simulink model "ADK_signal_transfer"  (R2021a)
settings: configuration reference "ADK_IDS_Speedgoat" (kept outside this file)
undefined symbols (not defined in the file): COMMUNICATION_CYCLE_TIME, desired_trajectory_index, GNSS_Status, h, km, m, MAX_LOCAL_TRAJECTORY_WAY_POINT_NUMBER, MAX_TRAJECTORY_WAY_POINT_NUMBER, O_ALTITUDE, O_LATITUDE, O_LONGITUDE, s
libraries: simulink x3, simulink_extras x2, aerolibconvert2 x1
settings Model: DataDictionary=ADK_IDS.sldd  Creator=xinrui  LastModifiedBy=Administrator
settings ConfigSetRef: SourceName=ADK_IDS_Speedgoat

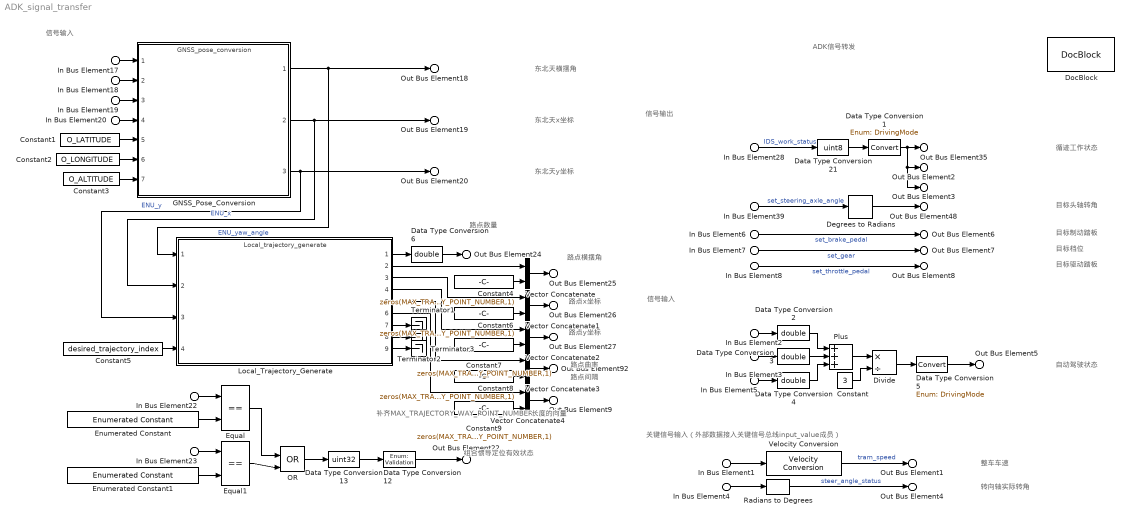
== system ADK_signal_transfer ==
  note: 信号输入
  note: 信号输出
  note: 信号输入
  note: 整车车速
  note: 关键信号输入（外部数据接入关键信号总线input_value成员）
  note: 转向轴实际转角
  note: 东北天横摆角
  note: 东北天x坐标
  note: 东北天y坐标
  note: 组合惯导定位有效状态
  note: 路点数量
  note: 路点横摆角
  note: 路点x坐标
  note: 路点y坐标
  note: 循迹工作状态
  note: 目标头轴转角
  note: 路点曲率
  note: 自动驾驶状态
  note: 目标制动踏板
  note: 目标档位
  note: 目标驱动踏板
  note: ADK信号转发
  note: 补齐MAX_TRAJECTORY_WAY_POINT_NUMBER长度的向量
  note: 路点间隔
  In Bus Element28 : Inport  PortName=IDS_InternalOutputPort  Element=IDS_work_status
  In Bus Element39 : Inport  PortName=IDS_InternalOutputPort  Element=steering_axle_info.set_angle.processed_value_current
  In Bus Element6 : Inport  PortName=IDS_InternalOutputPort  Element=AION_longitudinal_control_info.set_brake_pedal
  In Bus Element7 : Inport  PortName=IDS_InternalOutputPort  Element=AION_longitudinal_control_info.set_gear
  In Bus Element8 : Inport  PortName=IDS_InternalOutputPort  Element=AION_longitudinal_control_info.set_throttle_pedal
  In Bus Element2 : Inport  Port=2  PortName=IDS_InputPort  Element=InputCAN_bus.VCU2IDS_bus.VCU2IDS_brake_status.brake_pedal_enable_status
  In Bus Element1 : Inport  Port=2  PortName=IDS_InputPort  Element=InputCAN_bus.VCU2IDS_bus.VCU2IDS_status1.vehicle_speed
  In Bus Element3 : Inport  Port=2  PortName=IDS_InputPort  Element=InputCAN_bus.VCU2IDS_bus.VCU2IDS_steer_status.steer_angle_enable_status
  In Bus Element4 : Inport  Port=2  PortName=IDS_InputPort  Element=InputCAN_bus.VCU2IDS_bus.VCU2IDS_steer_status.steer_angle_status
  In Bus Element5 : Inport  Port=2  PortName=IDS_InputPort  Element=InputCAN_bus.VCU2IDS_bus.VCU2IDS_throttle_status.throttle_pedal_enable_status
  In Bus Element17 : Inport  Port=2  PortName=IDS_InputPort  Element=InputSerial_bus.GNSS2IDS_bus.Heading
  In Bus Element18 : Inport  Port=2  PortName=IDS_InputPort  Element=InputSerial_bus.GNSS2IDS_bus.Latitude
  In Bus Element19 : Inport  Port=2  PortName=IDS_InputPort  Element=InputSerial_bus.GNSS2IDS_bus.Longitude
  In Bus Element20 : Inport  Port=2  PortName=IDS_InputPort  Element=InputSerial_bus.GNSS2IDS_bus.Altitude
  In Bus Element22 : Inport  Port=2  PortName=IDS_InputPort  Element=InputSerial_bus.GNSS2IDS_bus.GNSSWorkStatus
  In Bus Element23 : Inport  Port=2  PortName=IDS_InputPort  Element=InputSerial_bus.GNSS2IDS_bus.GNSSWorkStatus
  Constant : Constant  Value=3
  Constant1 : Constant  Value=O_LATITUDE  OutDataTypeStr=double  SampleTime=COMMUNICATION_CYCLE_TIME
  Constant2 : Constant  Value=O_LONGITUDE  OutDataTypeStr=double  SampleTime=COMMUNICATION_CYCLE_TIME
  Constant3 : Constant  Value=O_ALTITUDE  OutDataTypeStr=double  SampleTime=COMMUNICATION_CYCLE_TIME
  Constant{4,6..9} (5 alike) : Constant  Value=zeros(MAX_TRAJECTORY_WAY_POINT_NUMBER - MAX_LOCAL_TRAJECTORY_WAY_POINT_NUMBER,1)  OutDataTypeStr=double  SampleTime=COMMUNICATION_CYCLE_TIME
  Constant5 : Constant  Value=desired_trajectory_index  OutDataTypeStr=int8  SampleTime=COMMUNICATION_CYCLE_TIME
  Data Type Conversion1 : DataTypeConversion  OutDataTypeStr=Enum: DrivingMode
  Data Type Conversion12 : DataTypeConversion  OutDataTypeStr=Enum: Validation
  Data Type Conversion13 : DataTypeConversion  OutDataTypeStr=uint32
  Data Type Conversion{2..4,6} (4 alike) : DataTypeConversion  OutDataTypeStr=double
  Data Type Conversion21 : DataTypeConversion  OutDataTypeStr=uint8
  Data Type Conversion5 : DataTypeConversion  OutDataTypeStr=Enum: DrivingMode
  Degrees to Radians : simulink_extras/Transformations/Degrees to Radians
  Divide : Product  Inputs=*/  OutDataTypeStr=uint8
  DocBlock : simulink/Model-Wide Utilities/DocBlock  DocumentType=HTML  mask(DocBlock){}
      mask Display:
      | plot([.8 0 0 1 1 .8 .8 1],[1 1 0 0 .8 1 .8 .8]);
      | text(.5,.6,'CHANGELOG','horizontalalignment','center');
      | text(.95,.05,get_param(gcb,'DocumentType'),'verticalalignment','bottom','horizontalalignment','right');
  Enumerated Constant : simulink/Sources/Enumerated Constant  OutDataTypeStr=Enum: GNSS_Status  Value=GNSS_Status.RTK_INT_Location  SampleTime=COMMUNICATION_CYCLE_TIME
  Enumerated Constant1 : simulink/Sources/Enumerated Constant  OutDataTypeStr=Enum: GNSS_Status  Value=GNSS_Status.RTK_INT_Orientation  SampleTime=COMMUNICATION_CYCLE_TIME
  Equal : RelationalOperator  Operator===  OutDataTypeStr=boolean  RndMeth=Simplest
  Equal1 : RelationalOperator  Operator===  OutDataTypeStr=boolean  RndMeth=Simplest
  GNSS_Pose_Conversion : ModelReference  ModelNameDialog=GNSS_pose_conversion  SimulationMode=Normal  ModelReferenceVersion=4.10
  Local_Trajectory_Generate : ModelReference  ModelNameDialog=Local_trajectory_generate.slx  SimulationMode=Normal  ModelReferenceVersion=1.200
  OR : Logic  Operator=OR  IconShape=distinctive  AllPortsSameDT=off  OutDataTypeStr=boolean
  Plus : Sum  Inputs=+++
  Radians to Degrees : simulink_extras/Transformations/Radians to Degrees
  Terminator1 : Terminator
  Terminator2 : Terminator
  Terminator3 : Terminator
  Vector Concatenate{,1..4} (5 alike) : Concatenate
  Velocity Conversion : aerolibconvert2/Velocity Conversion  IU=m/s  OU=km/h
  Out Bus Element1 : Outport  PortName=IDS_InternalInputPort  Element=tram_info.speed.input_value
  Out Bus Element5 : Outport  PortName=IDS_InternalInputPort  Element=tram_info.driving_mode
  Out Bus Element4 : Outport  PortName=IDS_InternalInputPort  Element=steering_axle_info.actual_angle.input_value
  Out Bus Element18 : Outport  PortName=IDS_InternalInputPort  Element=GNSS_info.ENU_yaw_angle
  Out Bus Element19 : Outport  PortName=IDS_InternalInputPort  Element=GNSS_info.ENU_x
  Out Bus Element20 : Outport  PortName=IDS_InternalInputPort  Element=GNSS_info.ENU_y
  Out Bus Element22 : Outport  PortName=IDS_InternalInputPort  Element=GNSS_info.location_valid_status
  Out Bus Element24 : Outport  PortName=IDS_InternalInputPort  Element=reference_trajectory_info.way_point_number
  Out Bus Element9 : Outport  PortName=IDS_InternalInputPort  Element=reference_trajectory_info.segment_length
  Out Bus Element25 : Outport  PortName=IDS_InternalInputPort  Element=reference_trajectory_info.trajectory_yaw_angle
  Out Bus Element26 : Outport  PortName=IDS_InternalInputPort  Element=reference_trajectory_info.trajectory_x
  Out Bus Element27 : Outport  PortName=IDS_InternalInputPort  Element=reference_trajectory_info.trajectory_y
  Out Bus Element92 : Outport  PortName=IDS_InternalInputPort  Element=reference_trajectory_info.trajectory_curvature
  Out Bus Element35 : Outport  Port=2  PortName=IDS_OuputPort  Element=OutputCAN_bus.IDS2VCU_bus.IDS2VCU_brake_command.brake_pedal_enable_command
  Out Bus Element6 : Outport  Port=2  PortName=IDS_OuputPort  Element=OutputCAN_bus.IDS2VCU_bus.IDS2VCU_brake_command.brake_pedal_command
  Out Bus Element7 : Outport  Port=2  PortName=IDS_OuputPort  Element=OutputCAN_bus.IDS2VCU_bus.IDS2VCU_gear_command.gear_command
  Out Bus Element2 : Outport  Port=2  PortName=IDS_OuputPort  Element=OutputCAN_bus.IDS2VCU_bus.IDS2VCU_steer_command.steer_angle_enable_command
  Out Bus Element48 : Outport  Port=2  PortName=IDS_OuputPort  Element=OutputCAN_bus.IDS2VCU_bus.IDS2VCU_steer_command.steer_angle_command
  Out Bus Element3 : Outport  Port=2  PortName=IDS_OuputPort  Element=OutputCAN_bus.IDS2VCU_bus.IDS2VCU_throttle_command.throttle_pedal_enable_command
  Out Bus Element8 : Outport  Port=2  PortName=IDS_OuputPort  Element=OutputCAN_bus.IDS2VCU_bus.IDS2VCU_throttle_command.throttle_pedal_command
  wires:
  In Bus Element17/1 -> GNSS_Pose_Conversion/1
  In Bus Element18/1 -> GNSS_Pose_Conversion/2
  In Bus Element19/1 -> GNSS_Pose_Conversion/3
  In Bus Element20/1 -> GNSS_Pose_Conversion/4
  Data Type Conversion13/1 -> Data Type Conversion12/1
  Enumerated Constant1/1 -> Equal1/2
  In Bus Element22/1 -> Equal/1
  In Bus Element23/1 -> Equal1/1
  Equal/1 -> OR/1
  OR/1 -> Data Type Conversion13/1
  Equal1/1 -> OR/2
  Enumerated Constant/1 -> Equal/2
  Data Type Conversion21/1 -> Data Type Conversion1/1
  Local_Trajectory_Generate/1 -> Data Type Conversion6/1
  Local_Trajectory_Generate/2 -> Vector Concatenate/1
  Local_Trajectory_Generate/3 -> Vector Concatenate1/1
  Local_Trajectory_Generate/4 -> Vector Concatenate2/1
  In Bus Element1/1 -> Velocity Conversion/1
  Velocity Conversion/1 -> Out Bus Element1/1  "tram_speed"
  In Bus Element4/1 -> Radians to Degrees/1
  In Bus Element39/1 -> Degrees to Radians/1  "set_steering_axle_angle"
  In Bus Element28/1 -> Data Type Conversion21/1  "IDS_work_status"
  Data Type Conversion12/1 -> Out Bus Element22/1
  Local_Trajectory_Generate/5 -> Vector Concatenate3/1
  Constant5/1 -> Local_Trajectory_Generate/4
  Data Type Conversion1/1 -> Out Bus Element35/1, Out Bus Element2/1, Out Bus Element3/1
  Degrees to Radians/1 -> Out Bus Element48/1
  In Bus Element2/1 -> Data Type Conversion2/1
  In Bus Element3/1 -> Data Type Conversion3/1
  In Bus Element5/1 -> Data Type Conversion4/1
  Data Type Conversion5/1 -> Out Bus Element5/1
  Data Type Conversion4/1 -> Plus/3
  Data Type Conversion3/1 -> Plus/2
  Data Type Conversion2/1 -> Plus/1
  Plus/1 -> Divide/1
  Constant/1 -> Divide/2
  Divide/1 -> Data Type Conversion5/1
  GNSS_Pose_Conversion/1 -> Out Bus Element18/1, Local_Trajectory_Generate/1  "ENU_yaw_angle"
  GNSS_Pose_Conversion/2 -> Out Bus Element19/1, Local_Trajectory_Generate/2  "ENU_x"
  GNSS_Pose_Conversion/3 -> Out Bus Element20/1, Local_Trajectory_Generate/3  "ENU_y"
  In Bus Element6/1 -> Out Bus Element6/1  "set_brake_pedal"
  In Bus Element7/1 -> Out Bus Element7/1  "set_gear"
  In Bus Element8/1 -> Out Bus Element8/1  "set_throttle_pedal"
  Constant2/1 -> GNSS_Pose_Conversion/6
  Constant3/1 -> GNSS_Pose_Conversion/7
  Constant1/1 -> GNSS_Pose_Conversion/5
  Radians to Degrees/1 -> Out Bus Element4/1  "steer_angle_status"
  Local_Trajectory_Generate/6 -> Vector Concatenate4/1
  Local_Trajectory_Generate/7 -> Terminator1/1
  Local_Trajectory_Generate/8 -> Terminator2/1
  Local_Trajectory_Generate/9 -> Terminator3/1
  Constant4/1 -> Vector Concatenate/2
  Vector Concatenate/1 -> Out Bus Element25/1
  Vector Concatenate1/1 -> Out Bus Element26/1
  Constant6/1 -> Vector Concatenate1/2
  Constant7/1 -> Vector Concatenate2/2
  Vector Concatenate2/1 -> Out Bus Element27/1
  Vector Concatenate3/1 -> Out Bus Element92/1
  Constant8/1 -> Vector Concatenate3/2
  Data Type Conversion6/1 -> Out Bus Element24/1
  Constant9/1 -> Vector Concatenate4/2
  Vector Concatenate4/1 -> Out Bus Element9/1
